simulink model "Ex2_3"  (R2016a)
settings: Solver=VariableStepAuto  StartTime=0.0  StopTime=10.0  RelTol=1e-3
settings Model: Creator=mende  LastModifiedBy=mende

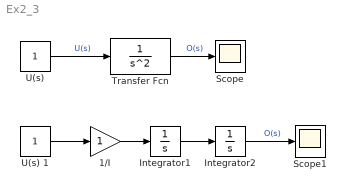
== system Ex2_3 ==
  1/I : Gain
  Integrator1 : Integrator
  Integrator2 : Integrator
  Scope : Scope
  Scope1 : Scope
  Transfer Fcn : TransferFcn  Denominator=[1 0 0]
  U(s) : Constant
  U(s) 1 : Constant
  wires:
  U(s)/1 -> Transfer Fcn/1  "U(s)"
  Transfer Fcn/1 -> Scope/1  "O(s)"
  U(s) 1/1 -> 1/I/1
  1/I/1 -> Integrator1/1
  Integrator1/1 -> Integrator2/1
  Integrator2/1 -> Scope1/1  "O(s)"
